simulink model "model_2_hardware"  (R2019b)
settings: Solver=VariableStepAuto  StartTime=0.0  StopTime=inf  RelTol=1e-3
values from neighbouring files (symbols this model uses):
  Cs = tf([c2 c1 c0], [1 0 0])    [params2.m]
  slope = (y2 - y1)/(x2 - x1)    (= 0.1)    [params2.m]
  y1 = 35    [params2.m]
libraries: arduinolib x2, simulink x2
settings Model: Creator=adityaaaap  LastModifiedBy=adityaaaap

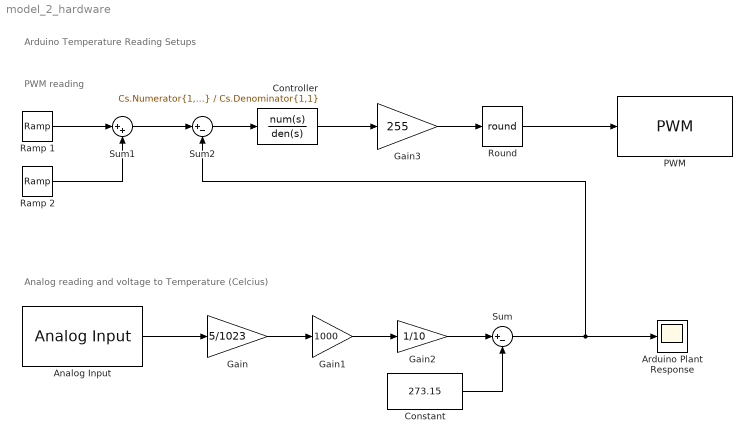
== system model_2_hardware ==
  note: Analog reading and voltage to Temperature (Celcius)
  note: Arduino Temperature Reading Setups
  note: PWM reading
  Analog Input : arduinolib/Analog Input  pinNumber=0  ReadResultsOnly=off  ConversionTriggerSource=Software  ExternalTriggerType=uint32(0)  OutputDataType=uint16  EnableConversionCompleteNotify=off  EnableOuputStatus=off  SampleTime=1  blockPlatform=arduino
  Arduino Plant Response : Scope
  Constant : Constant  Value=273.15
  Controller : TransferFcn  Numerator=Cs.Numerator{1,1}  Denominator=Cs.Denominator{1,1}
  Gain : Gain  Gain=5/1023
  Gain1 : Gain  Gain=1000
  Gain2 : Gain  Gain=1/10
  Gain3 : Gain  Gain=255
  PWM : arduinolib/PWM  pinNumber=7  EnableInputFrequency=off  InitialFrequency=2000  InitialDutyCycle=0  NotificationType=None  blockPlatform=arduino
  Ramp 1 : simulink/Sources/Ramp  slope=slope  start=x1  InitialOutput=0
  Ramp 2 : simulink/Sources/Ramp  slope=-slope  start=x2  InitialOutput=y1
  "Round " : Rounding  Operator=round
  Sum : Sum  Inputs=|+-
  Sum1 : Sum  Inputs=|++
  Sum2 : Sum  Inputs=|+-
  wires:
  Gain3/1 -> "Round "/1
  Analog Input/1 -> Gain/1
  Gain/1 -> Gain1/1
  Gain1/1 -> Gain2/1
  Constant/1 -> Sum/2
  Controller/1 -> Gain3/1
  Sum/1 -> Arduino Plant Response/1, Sum2/2
  Gain2/1 -> Sum/1
  "Round "/1 -> PWM/1
  Sum1/1 -> Sum2/1
  Sum2/1 -> Controller/1
  Ramp 2/1 -> Sum1/2
  Ramp 1/1 -> Sum1/1
